simulink model "altimeter"  (R2015a)
settings: Solver=ode45  StartTime=0.0  StopTime=10  RelTol=1e-3
undefined symbols (not defined in the file): altNoise, altOffset
libraries: simulink x1
settings Model: Creator=johnz  LastModifiedBy=johnz

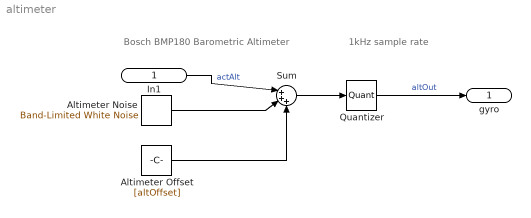
== system altimeter ==
  note: Bosch BMP180 Barometric Altimeter
  note: 1kHz sample rate
  In1 : Inport
  Altimeter Noise : simulink/Sources/Band-Limited White Noise  Cov=[altNoise]  Ts=1/1000  seed=[233419]
  Altimeter Offset : Constant  Value=[altOffset]
  Quantizer : Quantizer  QuantizationInterval=altSensitivity
  Sum : Sum  Inputs=|+++
  gyro : Outport  OutDataTypeStr=double  PortDimensions=1
  wires:
  In1/1 -> Sum/1  "actAlt"
  Sum/1 -> Quantizer/1
  Altimeter Offset/1 -> Sum/3
  Altimeter Noise/1 -> Sum/2
  Quantizer/1 -> gyro/1  "altOut"
